simulink model "VCU_CS75_12_27_test_log"  (R2014a)
settings: Solver=FixedStepDiscrete  StartTime=0.0  StopTime=25  FixedStep=0.0005  RelTol=1e-3
undefined symbols (not defined in the file or in its folder): ecucoder_acal, ErrorSumMax1, ErrorSumMax2, ErrorSumMax3, I1, I2, I3, I_SW01_L, LaterlAngleCommand, LDW, Log_ErrorSumMax1, Log_ErrorSumMax2, Log_I1, Log_I2, Log_P1, Log_P2, Log_Takeover, P1, P2, P3, RemoteAcc, RemoteAcclPosition
libraries: simulink x927, ec5744lib x40
(part 21 of 31)

== system VCU_CS75_12_27_test_log/长安CS75底盘程序，20ms一次/Output/Subsystem/TransmitMessages11/GW_LCDAL_2EA/LCDAL_SEAStatus ==
  LCDAL_SEAStatus : Inport
  Constant{1..2,4..8} (7 alike) : Constant  Value=0  OutDataTypeStr=uint8
  LCDAL_SEAStatusRon : Rounding  Operator=round
  LCDAL_SEAStatus_1sat : Saturate  UpperLimit=192  LowerLimit=0
  LCDAL_SEAStatus_Convert : DataTypeConversion  OutDataTypeStr=uint8
  LCDAL_SEAStatus_Convert1 : DataTypeConversion  OutDataTypeStr=uint32
  LCDAL_SEAStatus_D : Product  Inputs=*/
  LCDAL_SEAStatus_F : Constant  OutDataTypeStr=single
  LCDAL_SEAStatus_L : simulink/Logic and Bit Operations/Bitwise Operator  logicop=AND  UseBitMask=on  BitMask=192  BitMaskRealWorld=Stored Integer
  LCDAL_SEAStatus_O : Constant  Value=0  OutDataTypeStr=single
  LCDAL_SEAStatus_S : ArithShift  BitShiftNumber=-6
  LCDAL_SEAStatus_sat : Saturate  UpperLimit=3  LowerLimit=0
  LCDAL_SEAStatus_st : Sum  Inputs=+-
  output1 : Outport
  output2 : Outport  Port=2
  output3 : Outport  Port=3
  output4 : Outport  Port=4
  output5 : Outport  Port=5
  output6 : Outport  Port=6
  output7 : Outport  Port=7
  output8 : Outport  Port=8
  wires:
  Constant8/1 -> output8/1
  Constant7/1 -> output7/1
  Constant6/1 -> output6/1
  Constant5/1 -> output5/1
  Constant4/1 -> output4/1
  Constant2/1 -> output2/1
  Constant1/1 -> output1/1
  LCDAL_SEAStatus_Convert/1 -> output3/1
  LCDAL_SEAStatus_L/1 -> LCDAL_SEAStatus_Convert/1
  LCDAL_SEAStatus_Convert1/1 -> LCDAL_SEAStatus_L/1
  LCDAL_SEAStatus_1sat/1 -> LCDAL_SEAStatus_Convert1/1
  LCDAL_SEAStatus_S/1 -> LCDAL_SEAStatus_1sat/1
  LCDAL_SEAStatusRon/1 -> LCDAL_SEAStatus_S/1
  LCDAL_SEAStatus_D/1 -> LCDAL_SEAStatusRon/1
  LCDAL_SEAStatus_F/1 -> LCDAL_SEAStatus_D/2
  LCDAL_SEAStatus_st/1 -> LCDAL_SEAStatus_D/1
  LCDAL_SEAStatus_O/1 -> LCDAL_SEAStatus_st/2
  LCDAL_SEAStatus_sat/1 -> LCDAL_SEAStatus_st/1
  LCDAL_SEAStatus/1 -> LCDAL_SEAStatus_sat/1

== system VCU_CS75_12_27_test_log/长安CS75底盘程序，20ms一次/Output/Subsystem/TransmitMessages11/GW_LCDAL_2EA/LCDAL_SystemStatus ==
  LCDAL_SystemStatus : Inport
  Constant{1,3..8} (7 alike) : Constant  Value=0  OutDataTypeStr=uint8
  LCDAL_SystemStatusRon : Rounding  Operator=round
  LCDAL_SystemStatus_1sat : Saturate  UpperLimit=224  LowerLimit=0
  LCDAL_SystemStatus_Convert : DataTypeConversion  OutDataTypeStr=uint8
  LCDAL_SystemStatus_Convert1 : DataTypeConversion  OutDataTypeStr=uint32
  LCDAL_SystemStatus_D : Product  Inputs=*/
  LCDAL_SystemStatus_F : Constant  OutDataTypeStr=single
  LCDAL_SystemStatus_L : simulink/Logic and Bit Operations/Bitwise Operator  logicop=AND  UseBitMask=on  BitMask=224  BitMaskRealWorld=Stored Integer
  LCDAL_SystemStatus_O : Constant  Value=0  OutDataTypeStr=single
  LCDAL_SystemStatus_S : ArithShift  BitShiftNumber=-5
  LCDAL_SystemStatus_sat : Saturate  UpperLimit=7  LowerLimit=0
  LCDAL_SystemStatus_st : Sum  Inputs=+-
  output1 : Outport
  output2 : Outport  Port=2
  output3 : Outport  Port=3
  output4 : Outport  Port=4
  output5 : Outport  Port=5
  output6 : Outport  Port=6
  output7 : Outport  Port=7
  output8 : Outport  Port=8
  wires:
  Constant8/1 -> output8/1
  Constant7/1 -> output7/1
  Constant6/1 -> output6/1
  Constant5/1 -> output5/1
  Constant4/1 -> output4/1
  Constant3/1 -> output3/1
  Constant1/1 -> output1/1
  LCDAL_SystemStatus_Convert/1 -> output2/1
  LCDAL_SystemStatus_L/1 -> LCDAL_SystemStatus_Convert/1
  LCDAL_SystemStatus_Convert1/1 -> LCDAL_SystemStatus_L/1
  LCDAL_SystemStatus_1sat/1 -> LCDAL_SystemStatus_Convert1/1
  LCDAL_SystemStatus_S/1 -> LCDAL_SystemStatus_1sat/1
  LCDAL_SystemStatusRon/1 -> LCDAL_SystemStatus_S/1
  LCDAL_SystemStatus_D/1 -> LCDAL_SystemStatusRon/1
  LCDAL_SystemStatus_F/1 -> LCDAL_SystemStatus_D/2
  LCDAL_SystemStatus_st/1 -> LCDAL_SystemStatus_D/1
  LCDAL_SystemStatus_O/1 -> LCDAL_SystemStatus_st/2
  LCDAL_SystemStatus_sat/1 -> LCDAL_SystemStatus_st/1
  LCDAL_SystemStatus/1 -> LCDAL_SystemStatus_sat/1

== system VCU_CS75_12_27_test_log/长安CS75底盘程序，20ms一次/Output/Subsystem/TransmitMessages13/GW_LCDAR_2FA/LCDAR_BSDLCAAlert ==
  LCDAR_BSDLCAAlert : Inport
  Constant{2..8} (7 alike) : Constant  Value=0  OutDataTypeStr=uint8
  LCDAR_BSDLCAAlertRon : Rounding  Operator=round
  LCDAR_BSDLCAAlert_1sat : Saturate  UpperLimit=48  LowerLimit=0
  LCDAR_BSDLCAAlert_Convert : DataTypeConversion  OutDataTypeStr=uint8
  LCDAR_BSDLCAAlert_Convert1 : DataTypeConversion  OutDataTypeStr=uint32
  LCDAR_BSDLCAAlert_D : Product  Inputs=*/
  LCDAR_BSDLCAAlert_F : Constant  OutDataTypeStr=single
  LCDAR_BSDLCAAlert_L : simulink/Logic and Bit Operations/Bitwise Operator  logicop=AND  UseBitMask=on  BitMask=48  BitMaskRealWorld=Stored Integer
  LCDAR_BSDLCAAlert_O : Constant  Value=0  OutDataTypeStr=single
  LCDAR_BSDLCAAlert_S : ArithShift  BitShiftNumber=-4
  LCDAR_BSDLCAAlert_sat : Saturate  UpperLimit=3  LowerLimit=0
  LCDAR_BSDLCAAlert_st : Sum  Inputs=+-
  output1 : Outport
  output2 : Outport  Port=2
  output3 : Outport  Port=3
  output4 : Outport  Port=4
  output5 : Outport  Port=5
  output6 : Outport  Port=6
  output7 : Outport  Port=7
  output8 : Outport  Port=8
  wires:
  LCDAR_BSDLCAAlert/1 -> LCDAR_BSDLCAAlert_sat/1
  LCDAR_BSDLCAAlert_sat/1 -> LCDAR_BSDLCAAlert_st/1
  LCDAR_BSDLCAAlert_O/1 -> LCDAR_BSDLCAAlert_st/2
  LCDAR_BSDLCAAlert_st/1 -> LCDAR_BSDLCAAlert_D/1
  LCDAR_BSDLCAAlert_F/1 -> LCDAR_BSDLCAAlert_D/2
  LCDAR_BSDLCAAlert_D/1 -> LCDAR_BSDLCAAlertRon/1
  LCDAR_BSDLCAAlertRon/1 -> LCDAR_BSDLCAAlert_S/1
  LCDAR_BSDLCAAlert_S/1 -> LCDAR_BSDLCAAlert_1sat/1
  LCDAR_BSDLCAAlert_1sat/1 -> LCDAR_BSDLCAAlert_Convert1/1
  LCDAR_BSDLCAAlert_Convert1/1 -> LCDAR_BSDLCAAlert_L/1
  LCDAR_BSDLCAAlert_L/1 -> LCDAR_BSDLCAAlert_Convert/1
  LCDAR_BSDLCAAlert_Convert/1 -> output1/1
  Constant2/1 -> output2/1
  Constant3/1 -> output3/1
  Constant4/1 -> output4/1
  Constant5/1 -> output5/1
  Constant6/1 -> output6/1
  Constant7/1 -> output7/1
  Constant8/1 -> output8/1

== system VCU_CS75_12_27_test_log/长安CS75底盘程序，20ms一次/Output/Subsystem/TransmitMessages13/GW_LCDAR_2FA/LCDAR_BSDLCAStatus ==
  LCDAR_BSDLCAStatus : Inport
  Constant{1,3..8} (7 alike) : Constant  Value=0  OutDataTypeStr=uint8
  LCDAR_BSDLCAStatusRon : Rounding  Operator=round
  LCDAR_BSDLCAStatus_1sat : Saturate  UpperLimit=24  LowerLimit=0
  LCDAR_BSDLCAStatus_Convert : DataTypeConversion  OutDataTypeStr=uint8
  LCDAR_BSDLCAStatus_Convert1 : DataTypeConversion  OutDataTypeStr=uint32
  LCDAR_BSDLCAStatus_D : Product  Inputs=*/
  LCDAR_BSDLCAStatus_F : Constant  OutDataTypeStr=single
  LCDAR_BSDLCAStatus_L : simulink/Logic and Bit Operations/Bitwise Operator  logicop=AND  UseBitMask=on  BitMask=24  BitMaskRealWorld=Stored Integer
  LCDAR_BSDLCAStatus_O : Constant  Value=0  OutDataTypeStr=single
  LCDAR_BSDLCAStatus_S : ArithShift  BitShiftNumber=-3
  LCDAR_BSDLCAStatus_sat : Saturate  UpperLimit=3  LowerLimit=0
  LCDAR_BSDLCAStatus_st : Sum  Inputs=+-
  output1 : Outport
  output2 : Outport  Port=2
  output3 : Outport  Port=3
  output4 : Outport  Port=4
  output5 : Outport  Port=5
  output6 : Outport  Port=6
  output7 : Outport  Port=7
  output8 : Outport  Port=8
  wires:
  LCDAR_BSDLCAStatus/1 -> LCDAR_BSDLCAStatus_sat/1
  LCDAR_BSDLCAStatus_sat/1 -> LCDAR_BSDLCAStatus_st/1
  LCDAR_BSDLCAStatus_O/1 -> LCDAR_BSDLCAStatus_st/2
  LCDAR_BSDLCAStatus_st/1 -> LCDAR_BSDLCAStatus_D/1
  LCDAR_BSDLCAStatus_F/1 -> LCDAR_BSDLCAStatus_D/2
  LCDAR_BSDLCAStatus_D/1 -> LCDAR_BSDLCAStatusRon/1
  LCDAR_BSDLCAStatusRon/1 -> LCDAR_BSDLCAStatus_S/1
  LCDAR_BSDLCAStatus_S/1 -> LCDAR_BSDLCAStatus_1sat/1
  LCDAR_BSDLCAStatus_1sat/1 -> LCDAR_BSDLCAStatus_Convert1/1
  LCDAR_BSDLCAStatus_Convert1/1 -> LCDAR_BSDLCAStatus_L/1
  LCDAR_BSDLCAStatus_L/1 -> LCDAR_BSDLCAStatus_Convert/1
  LCDAR_BSDLCAStatus_Convert/1 -> output2/1
  Constant1/1 -> output1/1
  Constant3/1 -> output3/1
  Constant4/1 -> output4/1
  Constant5/1 -> output5/1
  Constant6/1 -> output6/1
  Constant7/1 -> output7/1
  Constant8/1 -> output8/1

== system VCU_CS75_12_27_test_log/长安CS75底盘程序，20ms一次/Output/Subsystem/TransmitMessages13/GW_LCDAR_2FA/LCDAR_CTAAlert ==
  LCDAR_CTAAlert : Inport
  Constant{2..8} (7 alike) : Constant  Value=0  OutDataTypeStr=uint8
  LCDAR_CTAAlertABS : Abs
  LCDAR_CTAAlertCS : ArithShift  BitShiftNumber=-2
  LCDAR_CTAAlertConS : Constant  OutDataTypeStr=single
  LCDAR_CTAAlertCosR : Constant  Value=0  OutDataTypeStr=uint8
  LCDAR_CTAAlertROP : RelationalOperator  Operator=<  OutDataTypeStr=boolean
  LCDAR_CTAAlertRon : Rounding  Operator=round
  LCDAR_CTAAlertSW : Switch  Criteria=u2 ~= 0
  LCDAR_CTAAlert_1sat : Saturate  UpperLimit=3  LowerLimit=0
  LCDAR_CTAAlert_Convert : DataTypeConversion  OutDataTypeStr=uint8
  LCDAR_CTAAlert_Convert1 : DataTypeConversion  OutDataTypeStr=uint32
  LCDAR_CTAAlert_D : Product  Inputs=*/
  LCDAR_CTAAlert_F : Constant  OutDataTypeStr=single
  LCDAR_CTAAlert_L : simulink/Logic and Bit Operations/Bitwise Operator  logicop=AND  UseBitMask=on  BitMask=3  BitMaskRealWorld=Stored Integer
  LCDAR_CTAAlert_O : Constant  Value=0  OutDataTypeStr=single
  LCDAR_CTAAlert_S : ArithShift
  LCDAR_CTAAlert_sat : Saturate  UpperLimit=3  LowerLimit=0
  LCDAR_CTAAlert_st : Sum  Inputs=+-
  LCDAR_CTAAlertsubcon : Sum  Inputs=+-
  output1 : Outport
  output2 : Outport  Port=2
  output3 : Outport  Port=3
  output4 : Outport  Port=4
  output5 : Outport  Port=5
  output6 : Outport  Port=6
  output7 : Outport  Port=7
  output8 : Outport  Port=8
  wires:
  LCDAR_CTAAlert/1 -> LCDAR_CTAAlert_sat/1
  LCDAR_CTAAlert_sat/1 -> LCDAR_CTAAlert_st/1
  LCDAR_CTAAlert_O/1 -> LCDAR_CTAAlert_st/2
  LCDAR_CTAAlert_st/1 -> LCDAR_CTAAlert_D/1
  LCDAR_CTAAlert_F/1 -> LCDAR_CTAAlert_D/2
  LCDAR_CTAAlert_D/1 -> LCDAR_CTAAlertRon/1
  LCDAR_CTAAlertRon/1 -> LCDAR_CTAAlertROP/1, LCDAR_CTAAlertABS/1, LCDAR_CTAAlertSW/3
  LCDAR_CTAAlertCosR/1 -> LCDAR_CTAAlertROP/2
  LCDAR_CTAAlertConS/1 -> LCDAR_CTAAlertCS/1
  LCDAR_CTAAlertCS/1 -> LCDAR_CTAAlertsubcon/1
  LCDAR_CTAAlertABS/1 -> LCDAR_CTAAlertsubcon/2
  LCDAR_CTAAlertsubcon/1 -> LCDAR_CTAAlertSW/1
  LCDAR_CTAAlertROP/1 -> LCDAR_CTAAlertSW/2
  LCDAR_CTAAlertSW/1 -> LCDAR_CTAAlert_S/1
  LCDAR_CTAAlert_S/1 -> LCDAR_CTAAlert_1sat/1
  LCDAR_CTAAlert_1sat/1 -> LCDAR_CTAAlert_Convert1/1
  LCDAR_CTAAlert_Convert1/1 -> LCDAR_CTAAlert_L/1
  LCDAR_CTAAlert_L/1 -> LCDAR_CTAAlert_Convert/1
  LCDAR_CTAAlert_Convert/1 -> output1/1
  Constant2/1 -> output2/1
  Constant3/1 -> output3/1
  Constant4/1 -> output4/1
  Constant5/1 -> output5/1
  Constant6/1 -> output6/1
  Constant7/1 -> output7/1
  Constant8/1 -> output8/1

== system VCU_CS75_12_27_test_log/长安CS75底盘程序，20ms一次/Output/Subsystem/TransmitMessages13/GW_LCDAR_2FA/LCDAR_CTAStatus ==
  LCDAR_CTAStatus : Inport
  Constant{1,3..8} (7 alike) : Constant  Value=0  OutDataTypeStr=uint8
  LCDAR_CTAStatusRon : Rounding  Operator=round
  LCDAR_CTAStatus_1sat : Saturate  UpperLimit=6  LowerLimit=0
  LCDAR_CTAStatus_Convert : DataTypeConversion  OutDataTypeStr=uint8
  LCDAR_CTAStatus_Convert1 : DataTypeConversion  OutDataTypeStr=uint32
  LCDAR_CTAStatus_D : Product  Inputs=*/
  LCDAR_CTAStatus_F : Constant  OutDataTypeStr=single
  LCDAR_CTAStatus_L : simulink/Logic and Bit Operations/Bitwise Operator  logicop=AND  UseBitMask=on  BitMask=6  BitMaskRealWorld=Stored Integer
  LCDAR_CTAStatus_O : Constant  Value=0  OutDataTypeStr=single
  LCDAR_CTAStatus_S : ArithShift  BitShiftNumber=-1
  LCDAR_CTAStatus_sat : Saturate  UpperLimit=3  LowerLimit=0
  LCDAR_CTAStatus_st : Sum  Inputs=+-
  output1 : Outport
  output2 : Outport  Port=2
  output3 : Outport  Port=3
  output4 : Outport  Port=4
  output5 : Outport  Port=5
  output6 : Outport  Port=6
  output7 : Outport  Port=7
  output8 : Outport  Port=8
  wires:
  LCDAR_CTAStatus/1 -> LCDAR_CTAStatus_sat/1
  LCDAR_CTAStatus_sat/1 -> LCDAR_CTAStatus_st/1
  LCDAR_CTAStatus_O/1 -> LCDAR_CTAStatus_st/2
  LCDAR_CTAStatus_st/1 -> LCDAR_CTAStatus_D/1
  LCDAR_CTAStatus_F/1 -> LCDAR_CTAStatus_D/2
  LCDAR_CTAStatus_D/1 -> LCDAR_CTAStatusRon/1
  LCDAR_CTAStatusRon/1 -> LCDAR_CTAStatus_S/1
  LCDAR_CTAStatus_S/1 -> LCDAR_CTAStatus_1sat/1
  LCDAR_CTAStatus_1sat/1 -> LCDAR_CTAStatus_Convert1/1
  LCDAR_CTAStatus_Convert1/1 -> LCDAR_CTAStatus_L/1
  LCDAR_CTAStatus_L/1 -> LCDAR_CTAStatus_Convert/1
  LCDAR_CTAStatus_Convert/1 -> output2/1
  Constant1/1 -> output1/1
  Constant3/1 -> output3/1
  Constant4/1 -> output4/1
  Constant5/1 -> output5/1
  Constant6/1 -> output6/1
  Constant7/1 -> output7/1
  Constant8/1 -> output8/1

== system VCU_CS75_12_27_test_log/长安CS75底盘程序，20ms一次/Output/Subsystem/TransmitMessages13/GW_LCDAR_2FA/LCDAR_RCWAlert ==
  LCDAR_RCWAlert : Inport
  Constant{1..2,4..8} (7 alike) : Constant  Value=0  OutDataTypeStr=uint8
  LCDAR_RCWAlertRon : Rounding  Operator=round
  LCDAR_RCWAlert_1sat : Saturate  UpperLimit=3  LowerLimit=0
  LCDAR_RCWAlert_Convert : DataTypeConversion  OutDataTypeStr=uint8
  LCDAR_RCWAlert_Convert1 : DataTypeConversion  OutDataTypeStr=uint32
  LCDAR_RCWAlert_D : Product  Inputs=*/
  LCDAR_RCWAlert_F : Constant  OutDataTypeStr=single
  LCDAR_RCWAlert_L : simulink/Logic and Bit Operations/Bitwise Operator  logicop=AND  UseBitMask=on  BitMask=3  BitMaskRealWorld=Stored Integer
  LCDAR_RCWAlert_O : Constant  Value=0  OutDataTypeStr=single
  LCDAR_RCWAlert_S : ArithShift
  LCDAR_RCWAlert_sat : Saturate  UpperLimit=3  LowerLimit=0
  LCDAR_RCWAlert_st : Sum  Inputs=+-
  output1 : Outport
  output2 : Outport  Port=2
  output3 : Outport  Port=3
  output4 : Outport  Port=4
  output5 : Outport  Port=5
  output6 : Outport  Port=6
  output7 : Outport  Port=7
  output8 : Outport  Port=8
  wires:
  LCDAR_RCWAlert/1 -> LCDAR_RCWAlert_sat/1
  LCDAR_RCWAlert_sat/1 -> LCDAR_RCWAlert_st/1
  LCDAR_RCWAlert_O/1 -> LCDAR_RCWAlert_st/2
  LCDAR_RCWAlert_st/1 -> LCDAR_RCWAlert_D/1
  LCDAR_RCWAlert_F/1 -> LCDAR_RCWAlert_D/2
  LCDAR_RCWAlert_D/1 -> LCDAR_RCWAlertRon/1
  LCDAR_RCWAlertRon/1 -> LCDAR_RCWAlert_S/1
  LCDAR_RCWAlert_S/1 -> LCDAR_RCWAlert_1sat/1
  LCDAR_RCWAlert_1sat/1 -> LCDAR_RCWAlert_Convert1/1
  LCDAR_RCWAlert_Convert1/1 -> LCDAR_RCWAlert_L/1
  LCDAR_RCWAlert_L/1 -> LCDAR_RCWAlert_Convert/1
  LCDAR_RCWAlert_Convert/1 -> output3/1
  Constant1/1 -> output1/1
  Constant2/1 -> output2/1
  Constant4/1 -> output4/1
  Constant5/1 -> output5/1
  Constant6/1 -> output6/1
  Constant7/1 -> output7/1
  Constant8/1 -> output8/1

== system VCU_CS75_12_27_test_log/长安CS75底盘程序，20ms一次/Output/Subsystem/TransmitMessages13/GW_LCDAR_2FA/LCDAR_RCWStatus ==
  LCDAR_RCWStatus : Inport
  Constant{1..3,5..8} (7 alike) : Constant  Value=0  OutDataTypeStr=uint8
  LCDAR_RCWStatusRon : Rounding  Operator=round
  LCDAR_RCWStatus_1sat : Saturate  UpperLimit=48  LowerLimit=0
  LCDAR_RCWStatus_Convert : DataTypeConversion  OutDataTypeStr=uint8
  LCDAR_RCWStatus_Convert1 : DataTypeConversion  OutDataTypeStr=uint32
  LCDAR_RCWStatus_D : Product  Inputs=*/
  LCDAR_RCWStatus_F : Constant  OutDataTypeStr=single
  LCDAR_RCWStatus_L : simulink/Logic and Bit Operations/Bitwise Operator  logicop=AND  UseBitMask=on  BitMask=48  BitMaskRealWorld=Stored Integer
  LCDAR_RCWStatus_O : Constant  Value=0  OutDataTypeStr=single
  LCDAR_RCWStatus_S : ArithShift  BitShiftNumber=-4
  LCDAR_RCWStatus_sat : Saturate  UpperLimit=3  LowerLimit=0
  LCDAR_RCWStatus_st : Sum  Inputs=+-
  output1 : Outport
  output2 : Outport  Port=2
  output3 : Outport  Port=3
  output4 : Outport  Port=4
  output5 : Outport  Port=5
  output6 : Outport  Port=6
  output7 : Outport  Port=7
  output8 : Outport  Port=8
  wires:
  LCDAR_RCWStatus/1 -> LCDAR_RCWStatus_sat/1
  LCDAR_RCWStatus_sat/1 -> LCDAR_RCWStatus_st/1
  LCDAR_RCWStatus_O/1 -> LCDAR_RCWStatus_st/2
  LCDAR_RCWStatus_st/1 -> LCDAR_RCWStatus_D/1
  LCDAR_RCWStatus_F/1 -> LCDAR_RCWStatus_D/2
  LCDAR_RCWStatus_D/1 -> LCDAR_RCWStatusRon/1
  LCDAR_RCWStatusRon/1 -> LCDAR_RCWStatus_S/1
  LCDAR_RCWStatus_S/1 -> LCDAR_RCWStatus_1sat/1
  LCDAR_RCWStatus_1sat/1 -> LCDAR_RCWStatus_Convert1/1
  LCDAR_RCWStatus_Convert1/1 -> LCDAR_RCWStatus_L/1
  LCDAR_RCWStatus_L/1 -> LCDAR_RCWStatus_Convert/1
  LCDAR_RCWStatus_Convert/1 -> output4/1
  Constant1/1 -> output1/1
  Constant2/1 -> output2/1
  Constant3/1 -> output3/1
  Constant5/1 -> output5/1
  Constant6/1 -> output6/1
  Constant7/1 -> output7/1
  Constant8/1 -> output8/1

== system VCU_CS75_12_27_test_log/长安CS75底盘程序，20ms一次/Output/Subsystem/TransmitMessages13/GW_LCDAR_2FA/LCDAR_SEAAlert ==
  LCDAR_SEAAlert : Inport
  Constant{2..8} (7 alike) : Constant  Value=0  OutDataTypeStr=uint8
  LCDAR_SEAAlertRon : Rounding  Operator=round
  LCDAR_SEAAlert_1sat : Saturate  UpperLimit=12  LowerLimit=0
  LCDAR_SEAAlert_Convert : DataTypeConversion  OutDataTypeStr=uint8
  LCDAR_SEAAlert_Convert1 : DataTypeConversion  OutDataTypeStr=uint32
  LCDAR_SEAAlert_D : Product  Inputs=*/
  LCDAR_SEAAlert_F : Constant  OutDataTypeStr=single
  LCDAR_SEAAlert_L : simulink/Logic and Bit Operations/Bitwise Operator  logicop=AND  UseBitMask=on  BitMask=12  BitMaskRealWorld=Stored Integer
  LCDAR_SEAAlert_O : Constant  Value=0  OutDataTypeStr=single
  LCDAR_SEAAlert_S : ArithShift  BitShiftNumber=-2
  LCDAR_SEAAlert_sat : Saturate  UpperLimit=3  LowerLimit=0
  LCDAR_SEAAlert_st : Sum  Inputs=+-
  output1 : Outport
  output2 : Outport  Port=2
  output3 : Outport  Port=3
  output4 : Outport  Port=4
  output5 : Outport  Port=5
  output6 : Outport  Port=6
  output7 : Outport  Port=7
  output8 : Outport  Port=8
  wires:
  LCDAR_SEAAlert/1 -> LCDAR_SEAAlert_sat/1
  LCDAR_SEAAlert_sat/1 -> LCDAR_SEAAlert_st/1
  LCDAR_SEAAlert_O/1 -> LCDAR_SEAAlert_st/2
  LCDAR_SEAAlert_st/1 -> LCDAR_SEAAlert_D/1
  LCDAR_SEAAlert_F/1 -> LCDAR_SEAAlert_D/2
  LCDAR_SEAAlert_D/1 -> LCDAR_SEAAlertRon/1
  LCDAR_SEAAlertRon/1 -> LCDAR_SEAAlert_S/1
  LCDAR_SEAAlert_S/1 -> LCDAR_SEAAlert_1sat/1
  LCDAR_SEAAlert_1sat/1 -> LCDAR_SEAAlert_Convert1/1
  LCDAR_SEAAlert_Convert1/1 -> LCDAR_SEAAlert_L/1
  LCDAR_SEAAlert_L/1 -> LCDAR_SEAAlert_Convert/1
  LCDAR_SEAAlert_Convert/1 -> output1/1
  Constant2/1 -> output2/1
  Constant3/1 -> output3/1
  Constant4/1 -> output4/1
  Constant5/1 -> output5/1
  Constant6/1 -> output6/1
  Constant7/1 -> output7/1
  Constant8/1 -> output8/1

== system VCU_CS75_12_27_test_log/长安CS75底盘程序，20ms一次/Output/Subsystem/TransmitMessages13/GW_LCDAR_2FA/LCDAR_SEAStatus ==
  LCDAR_SEAStatus : Inport
  Constant{1..2,4..8} (7 alike) : Constant  Value=0  OutDataTypeStr=uint8
  LCDAR_SEAStatusRon : Rounding  Operator=round
  LCDAR_SEAStatus_1sat : Saturate  UpperLimit=48  LowerLimit=0
  LCDAR_SEAStatus_Convert : DataTypeConversion  OutDataTypeStr=uint8
  LCDAR_SEAStatus_Convert1 : DataTypeConversion  OutDataTypeStr=uint32
  LCDAR_SEAStatus_D : Product  Inputs=*/
  LCDAR_SEAStatus_F : Constant  OutDataTypeStr=single
  LCDAR_SEAStatus_L : simulink/Logic and Bit Operations/Bitwise Operator  logicop=AND  UseBitMask=on  BitMask=48  BitMaskRealWorld=Stored Integer
  LCDAR_SEAStatus_O : Constant  Value=0  OutDataTypeStr=single
  LCDAR_SEAStatus_S : ArithShift  BitShiftNumber=-4
  LCDAR_SEAStatus_sat : Saturate  UpperLimit=3  LowerLimit=0
  LCDAR_SEAStatus_st : Sum  Inputs=+-
  output1 : Outport
  output2 : Outport  Port=2
  output3 : Outport  Port=3
  output4 : Outport  Port=4
  output5 : Outport  Port=5
  output6 : Outport  Port=6
  output7 : Outport  Port=7
  output8 : Outport  Port=8
  wires:
  LCDAR_SEAStatus/1 -> LCDAR_SEAStatus_sat/1
  LCDAR_SEAStatus_sat/1 -> LCDAR_SEAStatus_st/1
  LCDAR_SEAStatus_O/1 -> LCDAR_SEAStatus_st/2
  LCDAR_SEAStatus_st/1 -> LCDAR_SEAStatus_D/1
  LCDAR_SEAStatus_F/1 -> LCDAR_SEAStatus_D/2
  LCDAR_SEAStatus_D/1 -> LCDAR_SEAStatusRon/1
  LCDAR_SEAStatusRon/1 -> LCDAR_SEAStatus_S/1
  LCDAR_SEAStatus_S/1 -> LCDAR_SEAStatus_1sat/1
  LCDAR_SEAStatus_1sat/1 -> LCDAR_SEAStatus_Convert1/1
  LCDAR_SEAStatus_Convert1/1 -> LCDAR_SEAStatus_L/1
  LCDAR_SEAStatus_L/1 -> LCDAR_SEAStatus_Convert/1
  LCDAR_SEAStatus_Convert/1 -> output3/1
  Constant1/1 -> output1/1
  Constant2/1 -> output2/1
  Constant4/1 -> output4/1
  Constant5/1 -> output5/1
  Constant6/1 -> output6/1
  Constant7/1 -> output7/1
  Constant8/1 -> output8/1

== system VCU_CS75_12_27_test_log/长安CS75底盘程序，20ms一次/Output/Subsystem/TransmitMessages13/GW_LCDAR_2FA/LCDAR_SystemStatus ==
  LCDAR_SystemStatus : Inport
  Constant{1,3..8} (7 alike) : Constant  Value=0  OutDataTypeStr=uint8
  LCDAR_SystemStatusRon : Rounding  Operator=round
  LCDAR_SystemStatus_1sat : Saturate  UpperLimit=224  LowerLimit=0
  LCDAR_SystemStatus_Convert : DataTypeConversion  OutDataTypeStr=uint8
  LCDAR_SystemStatus_Convert1 : DataTypeConversion  OutDataTypeStr=uint32
  LCDAR_SystemStatus_D : Product  Inputs=*/
  LCDAR_SystemStatus_F : Constant  OutDataTypeStr=single
  LCDAR_SystemStatus_L : simulink/Logic and Bit Operations/Bitwise Operator  logicop=AND  UseBitMask=on  BitMask=224  BitMaskRealWorld=Stored Integer
  LCDAR_SystemStatus_O : Constant  Value=0  OutDataTypeStr=single
  LCDAR_SystemStatus_S : ArithShift  BitShiftNumber=-5
  LCDAR_SystemStatus_sat : Saturate  UpperLimit=7  LowerLimit=0
  LCDAR_SystemStatus_st : Sum  Inputs=+-
  output1 : Outport
  output2 : Outport  Port=2
  output3 : Outport  Port=3
  output4 : Outport  Port=4
  output5 : Outport  Port=5
  output6 : Outport  Port=6
  output7 : Outport  Port=7
  output8 : Outport  Port=8
  wires:
  LCDAR_SystemStatus/1 -> LCDAR_SystemStatus_sat/1
  LCDAR_SystemStatus_sat/1 -> LCDAR_SystemStatus_st/1
  LCDAR_SystemStatus_O/1 -> LCDAR_SystemStatus_st/2
  LCDAR_SystemStatus_st/1 -> LCDAR_SystemStatus_D/1
  LCDAR_SystemStatus_F/1 -> LCDAR_SystemStatus_D/2
  LCDAR_SystemStatus_D/1 -> LCDAR_SystemStatusRon/1
  LCDAR_SystemStatusRon/1 -> LCDAR_SystemStatus_S/1
  LCDAR_SystemStatus_S/1 -> LCDAR_SystemStatus_1sat/1
  LCDAR_SystemStatus_1sat/1 -> LCDAR_SystemStatus_Convert1/1
  LCDAR_SystemStatus_Convert1/1 -> LCDAR_SystemStatus_L/1
  LCDAR_SystemStatus_L/1 -> LCDAR_SystemStatus_Convert/1
  LCDAR_SystemStatus_Convert/1 -> output2/1
  Constant1/1 -> output1/1
  Constant3/1 -> output3/1
  Constant4/1 -> output4/1
  Constant5/1 -> output5/1
  Constant6/1 -> output6/1
  Constant7/1 -> output7/1
  Constant8/1 -> output8/1

== system VCU_CS75_12_27_test_log/长安CS75底盘程序，20ms一次/Output/Subsystem/TransmitMessages14/LAS_2AD/CRC ==
  CRC : Inport
  CRCRon : Rounding  Operator=round
  CRC_1sat : Saturate  UpperLimit=255  LowerLimit=0
  CRC_Convert : DataTypeConversion  OutDataTypeStr=uint8
  CRC_Convert1 : DataTypeConversion  OutDataTypeStr=uint32
  CRC_D : Product  Inputs=*/
  CRC_F : Constant  OutDataTypeStr=single
  CRC_L : simulink/Logic and Bit Operations/Bitwise Operator  logicop=AND  UseBitMask=on  BitMask=255  BitMaskRealWorld=Stored Integer
  CRC_O : Constant  Value=0  OutDataTypeStr=single
  CRC_S : ArithShift
  CRC_sat : Saturate  UpperLimit=0  LowerLimit=0
  CRC_st : Sum  Inputs=+-
  Constant{1..7} (7 alike) : Constant  Value=0  OutDataTypeStr=uint8
  output1 : Outport
  output2 : Outport  Port=2
  output3 : Outport  Port=3
  output4 : Outport  Port=4
  output5 : Outport  Port=5
  output6 : Outport  Port=6
  output7 : Outport  Port=7
  output8 : Outport  Port=8
  wires:
  Constant7/1 -> output7/1
  Constant6/1 -> output6/1
  Constant5/1 -> output5/1
  Constant4/1 -> output4/1
  Constant3/1 -> output3/1
  Constant2/1 -> output2/1
  Constant1/1 -> output1/1
  CRC_Convert/1 -> output8/1
  CRC_L/1 -> CRC_Convert/1
  CRC_Convert1/1 -> CRC_L/1
  CRC_1sat/1 -> CRC_Convert1/1
  CRC_S/1 -> CRC_1sat/1
  CRCRon/1 -> CRC_S/1
  CRC_D/1 -> CRCRon/1
  CRC_F/1 -> CRC_D/2
  CRC_st/1 -> CRC_D/1
  CRC_O/1 -> CRC_st/2
  CRC_sat/1 -> CRC_st/1
  CRC/1 -> CRC_sat/1

== system VCU_CS75_12_27_test_log/长安CS75底盘程序，20ms一次/Output/Subsystem/TransmitMessages14/LAS_2AD/LAS_DriverHandsOff ==
  LAS_DriverHandsOff : Inport
  Constant{1,3..8} (7 alike) : Constant  Value=0  OutDataTypeStr=uint8
  LAS_DriverHandsOffRon : Rounding  Operator=round
  LAS_DriverHandsOff_1sat : Saturate  UpperLimit=3  LowerLimit=0
  LAS_DriverHandsOff_Convert : DataTypeConversion  OutDataTypeStr=uint8
  LAS_DriverHandsOff_Convert1 : DataTypeConversion  OutDataTypeStr=uint32
  LAS_DriverHandsOff_D : Product  Inputs=*/
  LAS_DriverHandsOff_F : Constant  OutDataTypeStr=single
  LAS_DriverHandsOff_L : simulink/Logic and Bit Operations/Bitwise Operator  logicop=AND  UseBitMask=on  BitMask=3  BitMaskRealWorld=Stored Integer
  LAS_DriverHandsOff_O : Constant  Value=0  OutDataTypeStr=single
  LAS_DriverHandsOff_S : ArithShift
  LAS_DriverHandsOff_sat : Saturate  UpperLimit=3  LowerLimit=0
  LAS_DriverHandsOff_st : Sum  Inputs=+-
  output1 : Outport
  output2 : Outport  Port=2
  output3 : Outport  Port=3
  output4 : Outport  Port=4
  output5 : Outport  Port=5
  output6 : Outport  Port=6
  output7 : Outport  Port=7
  output8 : Outport  Port=8
  wires:
  Constant8/1 -> output8/1
  Constant7/1 -> output7/1
  Constant6/1 -> output6/1
  Constant5/1 -> output5/1
  Constant4/1 -> output4/1
  Constant3/1 -> output3/1
  Constant1/1 -> output1/1
  LAS_DriverHandsOff_Convert/1 -> output2/1
  LAS_DriverHandsOff_L/1 -> LAS_DriverHandsOff_Convert/1
  LAS_DriverHandsOff_Convert1/1 -> LAS_DriverHandsOff_L/1
  LAS_DriverHandsOff_1sat/1 -> LAS_DriverHandsOff_Convert1/1
  LAS_DriverHandsOff_S/1 -> LAS_DriverHandsOff_1sat/1
  LAS_DriverHandsOffRon/1 -> LAS_DriverHandsOff_S/1
  LAS_DriverHandsOff_D/1 -> LAS_DriverHandsOffRon/1
  LAS_DriverHandsOff_F/1 -> LAS_DriverHandsOff_D/2
  LAS_DriverHandsOff_st/1 -> LAS_DriverHandsOff_D/1
  LAS_DriverHandsOff_O/1 -> LAS_DriverHandsOff_st/2
  LAS_DriverHandsOff_sat/1 -> LAS_DriverHandsOff_st/1
  LAS_DriverHandsOff/1 -> LAS_DriverHandsOff_sat/1

== system VCU_CS75_12_27_test_log/长安CS75底盘程序，20ms一次/Output/Subsystem/TransmitMessages14/LAS_2AD/LAS_IACCMode ==
  LAS_IACCMode : Inport
  Constant{1..3,5..8} (7 alike) : Constant  Value=0  OutDataTypeStr=uint8
  LAS_IACCModeRon : Rounding  Operator=round
  LAS_IACCMode_1sat : Saturate  UpperLimit=7  LowerLimit=0
  LAS_IACCMode_Convert : DataTypeConversion  OutDataTypeStr=uint8
  LAS_IACCMode_Convert1 : DataTypeConversion  OutDataTypeStr=uint32
  LAS_IACCMode_D : Product  Inputs=*/
  LAS_IACCMode_F : Constant  OutDataTypeStr=single
  LAS_IACCMode_L : simulink/Logic and Bit Operations/Bitwise Operator  logicop=AND  UseBitMask=on  BitMask=7  BitMaskRealWorld=Stored Integer
  LAS_IACCMode_O : Constant  Value=0  OutDataTypeStr=single
  LAS_IACCMode_S : ArithShift
  LAS_IACCMode_sat : Saturate  UpperLimit=7  LowerLimit=0
  LAS_IACCMode_st : Sum  Inputs=+-
  output1 : Outport
  output2 : Outport  Port=2
  output3 : Outport  Port=3
  output4 : Outport  Port=4
  output5 : Outport  Port=5
  output6 : Outport  Port=6
  output7 : Outport  Port=7
  output8 : Outport  Port=8
  wires:
  Constant8/1 -> output8/1
  Constant7/1 -> output7/1
  Constant6/1 -> output6/1
  Constant5/1 -> output5/1
  Constant3/1 -> output3/1
  Constant2/1 -> output2/1
  Constant1/1 -> output1/1
  LAS_IACCMode_Convert/1 -> output4/1
  LAS_IACCMode_L/1 -> LAS_IACCMode_Convert/1
  LAS_IACCMode_Convert1/1 -> LAS_IACCMode_L/1
  LAS_IACCMode_1sat/1 -> LAS_IACCMode_Convert1/1
  LAS_IACCMode_S/1 -> LAS_IACCMode_1sat/1
  LAS_IACCModeRon/1 -> LAS_IACCMode_S/1
  LAS_IACCMode_D/1 -> LAS_IACCModeRon/1
  LAS_IACCMode_F/1 -> LAS_IACCMode_D/2
  LAS_IACCMode_st/1 -> LAS_IACCMode_D/1
  LAS_IACCMode_O/1 -> LAS_IACCMode_st/2
  LAS_IACCMode_sat/1 -> LAS_IACCMode_st/1
  LAS_IACCMode/1 -> LAS_IACCMode_sat/1

== system VCU_CS75_12_27_test_log/长安CS75底盘程序，20ms一次/Output/Subsystem/TransmitMessages14/LAS_2AD/LAS_IACCTextInfoForDriver ==
  LAS_IACCTextInfoForDriver : Inport
  Constant{1..3,5..8} (7 alike) : Constant  Value=0  OutDataTypeStr=uint8
  LAS_IACCTextInfoForDriverRon : Rounding  Operator=round
  LAS_IACCTextInfoForDriver_1sat : Saturate  UpperLimit=248  LowerLimit=0
  LAS_IACCTextInfoForDriver_Convert : DataTypeConversion  OutDataTypeStr=uint8
  LAS_IACCTextInfoForDriver_Convert1 : DataTypeConversion  OutDataTypeStr=uint32
  LAS_IACCTextInfoForDriver_D : Product  Inputs=*/
  LAS_IACCTextInfoForDriver_F : Constant  OutDataTypeStr=single
  LAS_IACCTextInfoForDriver_L : simulink/Logic and Bit Operations/Bitwise Operator  logicop=AND  UseBitMask=on  BitMask=248  BitMaskRealWorld=Stored Integer
  LAS_IACCTextInfoForDriver_O : Constant  Value=0  OutDataTypeStr=single
  LAS_IACCTextInfoForDriver_S : ArithShift  BitShiftNumber=-3
  LAS_IACCTextInfoForDriver_sat : Saturate  UpperLimit=0  LowerLimit=0
  LAS_IACCTextInfoForDriver_st : Sum  Inputs=+-
  output1 : Outport
  output2 : Outport  Port=2
  output3 : Outport  Port=3
  output4 : Outport  Port=4
  output5 : Outport  Port=5
  output6 : Outport  Port=6
  output7 : Outport  Port=7
  output8 : Outport  Port=8
  wires:
  Constant8/1 -> output8/1
  Constant7/1 -> output7/1
  Constant6/1 -> output6/1
  Constant5/1 -> output5/1
  Constant3/1 -> output3/1
  Constant2/1 -> output2/1
  Constant1/1 -> output1/1
  LAS_IACCTextInfoForDriver_Convert/1 -> output4/1
  LAS_IACCTextInfoForDriver_L/1 -> LAS_IACCTextInfoForDriver_Convert/1
  LAS_IACCTextInfoForDriver_Convert1/1 -> LAS_IACCTextInfoForDriver_L/1
  LAS_IACCTextInfoForDriver_1sat/1 -> LAS_IACCTextInfoForDriver_Convert1/1
  LAS_IACCTextInfoForDriver_S/1 -> LAS_IACCTextInfoForDriver_1sat/1
  LAS_IACCTextInfoForDriverRon/1 -> LAS_IACCTextInfoForDriver_S/1
  LAS_IACCTextInfoForDriver_D/1 -> LAS_IACCTextInfoForDriverRon/1
  LAS_IACCTextInfoForDriver_F/1 -> LAS_IACCTextInfoForDriver_D/2
  LAS_IACCTextInfoForDriver_st/1 -> LAS_IACCTextInfoForDriver_D/1
  LAS_IACCTextInfoForDriver_O/1 -> LAS_IACCTextInfoForDriver_st/2
  LAS_IACCTextInfoForDriver_sat/1 -> LAS_IACCTextInfoForDriver_st/1
  LAS_IACCTextInfoForDriver/1 -> LAS_IACCTextInfoForDriver_sat/1

== system VCU_CS75_12_27_test_log/长安CS75底盘程序，20ms一次/Output/Subsystem/TransmitMessages14/LAS_2AD/LAS_TargetBasedLateralCOntrol ==
  LAS_TargetBasedLateralCOntrol : Inport
  Constant{2..8} (7 alike) : Constant  Value=0  OutDataTypeStr=uint8
  LAS_TargetBasedLateralCOntrolRon : Rounding  Operator=round
  LAS_TargetBasedLateralCOntrol_1sat : Saturate  UpperLimit=3  LowerLimit=0
  LAS_TargetBasedLateralCOntrol_Convert : DataTypeConversion  OutDataTypeStr=uint8
  LAS_TargetBasedLateralCOntrol_Convert1 : DataTypeConversion  OutDataTypeStr=uint32
  LAS_TargetBasedLateralCOntrol_D : Product  Inputs=*/
  LAS_TargetBasedLateralCOntrol_F : Constant  OutDataTypeStr=single
  LAS_TargetBasedLateralCOntrol_L : simulink/Logic and Bit Operations/Bitwise Operator  logicop=AND  UseBitMask=on  BitMask=3  BitMaskRealWorld=Stored Integer
  LAS_TargetBasedLateralCOntrol_O : Constant  Value=0  OutDataTypeStr=single
  LAS_TargetBasedLateralCOntrol_S : ArithShift
  LAS_TargetBasedLateralCOntrol_sat : Saturate  UpperLimit=0  LowerLimit=0
  LAS_TargetBasedLateralCOntrol_st : Sum  Inputs=+-
  output1 : Outport
  output2 : Outport  Port=2
  output3 : Outport  Port=3
  output4 : Outport  Port=4
  output5 : Outport  Port=5
  output6 : Outport  Port=6
  output7 : Outport  Port=7
  output8 : Outport  Port=8
  wires:
  Constant8/1 -> output8/1
  Constant7/1 -> output7/1
  Constant6/1 -> output6/1
  Constant5/1 -> output5/1
  Constant4/1 -> output4/1
  Constant3/1 -> output3/1
  Constant2/1 -> output2/1
  LAS_TargetBasedLateralCOntrol_Convert/1 -> output1/1
  LAS_TargetBasedLateralCOntrol_L/1 -> LAS_TargetBasedLateralCOntrol_Convert/1
  LAS_TargetBasedLateralCOntrol_Convert1/1 -> LAS_TargetBasedLateralCOntrol_L/1
  LAS_TargetBasedLateralCOntrol_1sat/1 -> LAS_TargetBasedLateralCOntrol_Convert1/1
  LAS_TargetBasedLateralCOntrol_S/1 -> LAS_TargetBasedLateralCOntrol_1sat/1
  LAS_TargetBasedLateralCOntrolRon/1 -> LAS_TargetBasedLateralCOntrol_S/1
  LAS_TargetBasedLateralCOntrol_D/1 -> LAS_TargetBasedLateralCOntrolRon/1
  LAS_TargetBasedLateralCOntrol_F/1 -> LAS_TargetBasedLateralCOntrol_D/2
  LAS_TargetBasedLateralCOntrol_st/1 -> LAS_TargetBasedLateralCOntrol_D/1
  LAS_TargetBasedLateralCOntrol_O/1 -> LAS_TargetBasedLateralCOntrol_st/2
  LAS_TargetBasedLateralCOntrol_sat/1 -> LAS_TargetBasedLateralCOntrol_st/1
  LAS_TargetBasedLateralCOntrol/1 -> LAS_TargetBasedLateralCOntrol_sat/1

== system VCU_CS75_12_27_test_log/长安CS75底盘程序，20ms一次/Output/Subsystem/TransmitMessages14/LAS_2AD/RollingConter ==
  RollingConter : Inport
  Constant{1..6,8} (7 alike) : Constant  Value=0  OutDataTypeStr=uint8
  RollingConterRon : Rounding  Operator=round
  RollingConter_1sat : Saturate  UpperLimit=15  LowerLimit=0
  RollingConter_Convert : DataTypeConversion  OutDataTypeStr=uint8
  RollingConter_Convert1 : DataTypeConversion  OutDataTypeStr=uint32
  RollingConter_D : Product  Inputs=*/
  RollingConter_F : Constant  OutDataTypeStr=single
  RollingConter_L : simulink/Logic and Bit Operations/Bitwise Operator  logicop=AND  UseBitMask=on  BitMask=15  BitMaskRealWorld=Stored Integer
  RollingConter_O : Constant  Value=0  OutDataTypeStr=single
  RollingConter_S : ArithShift
  RollingConter_sat : Saturate  UpperLimit=0  LowerLimit=0
  RollingConter_st : Sum  Inputs=+-
  output1 : Outport
  output2 : Outport  Port=2
  output3 : Outport  Port=3
  output4 : Outport  Port=4
  output5 : Outport  Port=5
  output6 : Outport  Port=6
  output7 : Outport  Port=7
  output8 : Outport  Port=8
  wires:
  Constant8/1 -> output8/1
  Constant6/1 -> output6/1
  Constant5/1 -> output5/1
  Constant4/1 -> output4/1
  Constant3/1 -> output3/1
  Constant2/1 -> output2/1
  Constant1/1 -> output1/1
  RollingConter_Convert/1 -> output7/1
  RollingConter_L/1 -> RollingConter_Convert/1
  RollingConter_Convert1/1 -> RollingConter_L/1
  RollingConter_1sat/1 -> RollingConter_Convert1/1
  RollingConter_S/1 -> RollingConter_1sat/1
  RollingConterRon/1 -> RollingConter_S/1
  RollingConter_D/1 -> RollingConterRon/1
  RollingConter_F/1 -> RollingConter_D/2
  RollingConter_st/1 -> RollingConter_D/1
  RollingConter_O/1 -> RollingConter_st/2
  RollingConter_sat/1 -> RollingConter_st/1
  RollingConter/1 -> RollingConter_sat/1

== system VCU_CS75_12_27_test_log/长安CS75底盘程序，20ms一次/Output/Subsystem/TransmitMessages2/ACC_3C5/ACC_TargetRange ==
  ACC_TargetRange : Inport
  ACC_TargetRangeBitCov : DataTypeConversion  OutDataTypeStr=uint8
  ACC_TargetRangeCOV : DataTypeConversion  OutDataTypeStr=uint8
  ACC_TargetRangeRon : Rounding  Operator=round
  ACC_TargetRange_1sat : Saturate  UpperLimit=65408  LowerLimit=0
  ACC_TargetRange_And : simulink/Logic and Bit Operations/Bitwise Operator  logicop=AND  UseBitMask=off  NumInputPorts=2  BitMask=bin2dec('11011001')  BitMaskRealWorld=Stored Integer
  ACC_TargetRange_And_C : Constant  Value=255  OutDataTypeStr=uint32
  ACC_TargetRange_Convert : DataTypeConversion  OutDataTypeStr=uint32
  ACC_TargetRange_D : Product  Inputs=*/
  ACC_TargetRange_D1 : Product  Inputs=*/
  ACC_TargetRange_F : Constant  Value=0.5  OutDataTypeStr=single
  ACC_TargetRange_L : simulink/Logic and Bit Operations/Bitwise Operator  logicop=AND  UseBitMask=on  BitMask=65408  BitMaskRealWorld=Stored Integer
  ACC_TargetRange_O : Constant  Value=0  OutDataTypeStr=single
  ACC_TargetRange_S : ArithShift  BitShiftNumber=-7
  ACC_TargetRange_sat : Saturate  UpperLimit=250  LowerLimit=0
  ACC_TargetRange_st : Sum  Inputs=+-
  ACC_TargetRangeoutput2_C : Constant  Value=256
  Constant{1,4..8} (6 alike) : Constant  Value=0  OutDataTypeStr=uint8
  output1 : Outport
  output2 : Outport  Port=2
  output3 : Outport  Port=3
  output4 : Outport  Port=4
  output5 : Outport  Port=5
  output6 : Outport  Port=6
  output7 : Outport  Port=7
  output8 : Outport  Port=8
  wires:
  ACC_TargetRange/1 -> ACC_TargetRange_sat/1
  ACC_TargetRange_sat/1 -> ACC_TargetRange_st/1
  ACC_TargetRange_O/1 -> ACC_TargetRange_st/2
  ACC_TargetRange_st/1 -> ACC_TargetRange_D/1
  ACC_TargetRange_F/1 -> ACC_TargetRange_D/2
  ACC_TargetRange_D/1 -> ACC_TargetRangeRon/1
  ACC_TargetRangeRon/1 -> ACC_TargetRange_S/1
  ACC_TargetRange_S/1 -> ACC_TargetRange_1sat/1
  ACC_TargetRange_1sat/1 -> ACC_TargetRange_Convert/1
  ACC_TargetRange_Convert/1 -> ACC_TargetRange_L/1
  ACC_TargetRange_L/1 -> ACC_TargetRange_D1/1, ACC_TargetRange_And/1
  ACC_TargetRangeoutput2_C/1 -> ACC_TargetRange_D1/2
  ACC_TargetRange_D1/1 -> ACC_TargetRangeCOV/1
  ACC_TargetRangeCOV/1 -> output2/1
  ACC_TargetRange_And_C/1 -> ACC_TargetRange_And/2
  ACC_TargetRange_And/1 -> ACC_TargetRangeBitCov/1
  ACC_TargetRangeBitCov/1 -> output3/1
  Constant1/1 -> output1/1
  Constant4/1 -> output4/1
  Constant5/1 -> output5/1
  Constant6/1 -> output6/1
  Constant7/1 -> output7/1
  Constant8/1 -> output8/1

== system VCU_CS75_12_27_test_log/长安CS75底盘程序，20ms一次/Output/Subsystem/TransmitMessages2/ACC_3C5/ACC_TargetType ==
  ACC_TargetType : Inport
  ACC_TargetTypeRon : Rounding  Operator=round
  ACC_TargetType_1sat : Saturate  UpperLimit=7  LowerLimit=0
  ACC_TargetType_Convert : DataTypeConversion  OutDataTypeStr=uint8
  ACC_TargetType_Convert1 : DataTypeConversion  OutDataTypeStr=uint32
  ACC_TargetType_D : Product  Inputs=*/
  ACC_TargetType_F : Constant  OutDataTypeStr=single
  ACC_TargetType_L : simulink/Logic and Bit Operations/Bitwise Operator  logicop=AND  UseBitMask=on  BitMask=7  BitMaskRealWorld=Stored Integer
  ACC_TargetType_O : Constant  Value=0  OutDataTypeStr=single
  ACC_TargetType_S : ArithShift
  ACC_TargetType_sat : Saturate  UpperLimit=0  LowerLimit=0
  ACC_TargetType_st : Sum  Inputs=+-
  Constant{1..3,5..8} (7 alike) : Constant  Value=0  OutDataTypeStr=uint8
  output1 : Outport
  output2 : Outport  Port=2
  output3 : Outport  Port=3
  output4 : Outport  Port=4
  output5 : Outport  Port=5
  output6 : Outport  Port=6
  output7 : Outport  Port=7
  output8 : Outport  Port=8
  wires:
  ACC_TargetType/1 -> ACC_TargetType_sat/1
  ACC_TargetType_sat/1 -> ACC_TargetType_st/1
  ACC_TargetType_O/1 -> ACC_TargetType_st/2
  ACC_TargetType_st/1 -> ACC_TargetType_D/1
  ACC_TargetType_F/1 -> ACC_TargetType_D/2
  ACC_TargetType_D/1 -> ACC_TargetTypeRon/1
  ACC_TargetTypeRon/1 -> ACC_TargetType_S/1
  ACC_TargetType_S/1 -> ACC_TargetType_1sat/1
  ACC_TargetType_1sat/1 -> ACC_TargetType_Convert1/1
  ACC_TargetType_Convert1/1 -> ACC_TargetType_L/1
  ACC_TargetType_L/1 -> ACC_TargetType_Convert/1
  ACC_TargetType_Convert/1 -> output4/1
  Constant1/1 -> output1/1
  Constant2/1 -> output2/1
  Constant3/1 -> output3/1
  Constant5/1 -> output5/1
  Constant6/1 -> output6/1
  Constant7/1 -> output7/1
  Constant8/1 -> output8/1

== system VCU_CS75_12_27_test_log/长安CS75底盘程序，20ms一次/Output/Subsystem/TransmitMessages2/ACC_3C5/CRC ==
  CRC : Inport
  CRCRon : Rounding  Operator=round
  CRC_1sat : Saturate  UpperLimit=255  LowerLimit=0
  CRC_Convert : DataTypeConversion  OutDataTypeStr=uint8
  CRC_Convert1 : DataTypeConversion  OutDataTypeStr=uint32
  CRC_D : Product  Inputs=*/
  CRC_F : Constant  OutDataTypeStr=single
  CRC_L : simulink/Logic and Bit Operations/Bitwise Operator  logicop=AND  UseBitMask=on  BitMask=255  BitMaskRealWorld=Stored Integer
  CRC_O : Constant  Value=0  OutDataTypeStr=single
  CRC_S : ArithShift
  CRC_sat : Saturate  UpperLimit=0  LowerLimit=0
  CRC_st : Sum  Inputs=+-
  Constant{1..7} (7 alike) : Constant  Value=0  OutDataTypeStr=uint8
  output1 : Outport
  output2 : Outport  Port=2
  output3 : Outport  Port=3
  output4 : Outport  Port=4
  output5 : Outport  Port=5
  output6 : Outport  Port=6
  output7 : Outport  Port=7
  output8 : Outport  Port=8
  wires:
  CRC/1 -> CRC_sat/1
  CRC_sat/1 -> CRC_st/1
  CRC_O/1 -> CRC_st/2
  CRC_st/1 -> CRC_D/1
  CRC_F/1 -> CRC_D/2
  CRC_D/1 -> CRCRon/1
  CRCRon/1 -> CRC_S/1
  CRC_S/1 -> CRC_1sat/1
  CRC_1sat/1 -> CRC_Convert1/1
  CRC_Convert1/1 -> CRC_L/1
  CRC_L/1 -> CRC_Convert/1
  CRC_Convert/1 -> output8/1
  Constant1/1 -> output1/1
  Constant2/1 -> output2/1
  Constant3/1 -> output3/1
  Constant4/1 -> output4/1
  Constant5/1 -> output5/1
  Constant6/1 -> output6/1
  Constant7/1 -> output7/1

== system VCU_CS75_12_27_test_log/长安CS75底盘程序，20ms一次/Output/Subsystem/TransmitMessages2/ACC_3C5/RollingConter ==
  RollingConter : Inport
  Constant{1..6,8} (7 alike) : Constant  Value=0  OutDataTypeStr=uint8
  RollingConterRon : Rounding  Operator=round
  RollingConter_1sat : Saturate  UpperLimit=15  LowerLimit=0
  RollingConter_Convert : DataTypeConversion  OutDataTypeStr=uint8
  RollingConter_Convert1 : DataTypeConversion  OutDataTypeStr=uint32
  RollingConter_D : Product  Inputs=*/
  RollingConter_F : Constant  OutDataTypeStr=single
  RollingConter_L : simulink/Logic and Bit Operations/Bitwise Operator  logicop=AND  UseBitMask=on  BitMask=15  BitMaskRealWorld=Stored Integer
  RollingConter_O : Constant  Value=0  OutDataTypeStr=single
  RollingConter_S : ArithShift
  RollingConter_sat : Saturate  UpperLimit=15  LowerLimit=0
  RollingConter_st : Sum  Inputs=+-
  output1 : Outport
  output2 : Outport  Port=2
  output3 : Outport  Port=3
  output4 : Outport  Port=4
  output5 : Outport  Port=5
  output6 : Outport  Port=6
  output7 : Outport  Port=7
  output8 : Outport  Port=8
  wires:
  RollingConter/1 -> RollingConter_sat/1
  RollingConter_sat/1 -> RollingConter_st/1
  RollingConter_O/1 -> RollingConter_st/2
  RollingConter_st/1 -> RollingConter_D/1
  RollingConter_F/1 -> RollingConter_D/2
  RollingConter_D/1 -> RollingConterRon/1
  RollingConterRon/1 -> RollingConter_S/1
  RollingConter_S/1 -> RollingConter_1sat/1
  RollingConter_1sat/1 -> RollingConter_Convert1/1
  RollingConter_Convert1/1 -> RollingConter_L/1
  RollingConter_L/1 -> RollingConter_Convert/1
  RollingConter_Convert/1 -> output7/1
  Constant1/1 -> output1/1
  Constant2/1 -> output2/1
  Constant3/1 -> output3/1
  Constant4/1 -> output4/1
  Constant5/1 -> output5/1
  Constant6/1 -> output6/1
  Constant8/1 -> output8/1

== system VCU_CS75_12_27_test_log/长安CS75底盘程序，20ms一次/Output/Subsystem/TransmitMessages3/ACC_3D5/ACC_LeftTargetDection ==
  ACC_LeftTargetDection : Inport
  ACC_LeftTargetDectionRon : Rounding  Operator=round
  ACC_LeftTargetDection_1sat : Saturate  UpperLimit=24  LowerLimit=0
  ACC_LeftTargetDection_Convert : DataTypeConversion  OutDataTypeStr=uint8
  ACC_LeftTargetDection_Convert1 : DataTypeConversion  OutDataTypeStr=uint32
  ACC_LeftTargetDection_D : Product  Inputs=*/
  ACC_LeftTargetDection_F : Constant  OutDataTypeStr=single
  ACC_LeftTargetDection_L : simulink/Logic and Bit Operations/Bitwise Operator  logicop=AND  UseBitMask=on  BitMask=24  BitMaskRealWorld=Stored Integer
  ACC_LeftTargetDection_O : Constant  Value=0  OutDataTypeStr=single
  ACC_LeftTargetDection_S : ArithShift  BitShiftNumber=-3
  ACC_LeftTargetDection_sat : Saturate  UpperLimit=0  LowerLimit=0
  ACC_LeftTargetDection_st : Sum  Inputs=+-
  Constant{2..8} (7 alike) : Constant  Value=0  OutDataTypeStr=uint8
  output1 : Outport
  output2 : Outport  Port=2
  output3 : Outport  Port=3
  output4 : Outport  Port=4
  output5 : Outport  Port=5
  output6 : Outport  Port=6
  output7 : Outport  Port=7
  output8 : Outport  Port=8
  wires:
  ACC_LeftTargetDection/1 -> ACC_LeftTargetDection_sat/1
  ACC_LeftTargetDection_sat/1 -> ACC_LeftTargetDection_st/1
  ACC_LeftTargetDection_O/1 -> ACC_LeftTargetDection_st/2
  ACC_LeftTargetDection_st/1 -> ACC_LeftTargetDection_D/1
  ACC_LeftTargetDection_F/1 -> ACC_LeftTargetDection_D/2
  ACC_LeftTargetDection_D/1 -> ACC_LeftTargetDectionRon/1
  ACC_LeftTargetDectionRon/1 -> ACC_LeftTargetDection_S/1
  ACC_LeftTargetDection_S/1 -> ACC_LeftTargetDection_1sat/1
  ACC_LeftTargetDection_1sat/1 -> ACC_LeftTargetDection_Convert1/1
  ACC_LeftTargetDection_Convert1/1 -> ACC_LeftTargetDection_L/1
  ACC_LeftTargetDection_L/1 -> ACC_LeftTargetDection_Convert/1
  ACC_LeftTargetDection_Convert/1 -> output1/1
  Constant2/1 -> output2/1
  Constant3/1 -> output3/1
  Constant4/1 -> output4/1
  Constant5/1 -> output5/1
  Constant6/1 -> output6/1
  Constant7/1 -> output7/1
  Constant8/1 -> output8/1

== system VCU_CS75_12_27_test_log/长安CS75底盘程序，20ms一次/Output/Subsystem/TransmitMessages3/ACC_3D5/ACC_LeftTargetLatRange ==
  ACC_LeftTargetLatRange : Inport
  ACC_LeftTargetLatRangeBitCov : DataTypeConversion  OutDataTypeStr=uint8
  ACC_LeftTargetLatRangeCOV : DataTypeConversion  OutDataTypeStr=uint8
  ACC_LeftTargetLatRangeRon : Rounding  Operator=round
  ACC_LeftTargetLatRange_1sat : Saturate  UpperLimit=8184  LowerLimit=0
  ACC_LeftTargetLatRange_And : simulink/Logic and Bit Operations/Bitwise Operator  logicop=AND  UseBitMask=off  NumInputPorts=2  BitMask=bin2dec('11011001')  BitMaskRealWorld=Stored Integer
  ACC_LeftTargetLatRange_And_C : Constant  Value=255  OutDataTypeStr=uint32
  ACC_LeftTargetLatRange_Convert : DataTypeConversion  OutDataTypeStr=uint32
  ACC_LeftTargetLatRange_D : Product  Inputs=*/
  ACC_LeftTargetLatRange_D1 : Product  Inputs=*/
  ACC_LeftTargetLatRange_F : Constant  Value=0.1  OutDataTypeStr=single
  ACC_LeftTargetLatRange_L : simulink/Logic and Bit Operations/Bitwise Operator  logicop=AND  UseBitMask=on  BitMask=8184  BitMaskRealWorld=Stored Integer
  ACC_LeftTargetLatRange_O : Constant  Value=-50  OutDataTypeStr=single
  ACC_LeftTargetLatRange_S : ArithShift  BitShiftNumber=-3
  ACC_LeftTargetLatRange_sat : Saturate  UpperLimit=0  LowerLimit=0
  ACC_LeftTargetLatRange_st : Sum  Inputs=+-
  ACC_LeftTargetLatRangeoutput3_C : Constant  Value=256
  Constant{1..2,5..8} (6 alike) : Constant  Value=0  OutDataTypeStr=uint8
  output1 : Outport
  output2 : Outport  Port=2
  output3 : Outport  Port=3
  output4 : Outport  Port=4
  output5 : Outport  Port=5
  output6 : Outport  Port=6
  output7 : Outport  Port=7
  output8 : Outport  Port=8
  wires:
  ACC_LeftTargetLatRange/1 -> ACC_LeftTargetLatRange_sat/1
  ACC_LeftTargetLatRange_sat/1 -> ACC_LeftTargetLatRange_st/1
  ACC_LeftTargetLatRange_O/1 -> ACC_LeftTargetLatRange_st/2
  ACC_LeftTargetLatRange_st/1 -> ACC_LeftTargetLatRange_D/1
  ACC_LeftTargetLatRange_F/1 -> ACC_LeftTargetLatRange_D/2
  ACC_LeftTargetLatRange_D/1 -> ACC_LeftTargetLatRangeRon/1
  ACC_LeftTargetLatRangeRon/1 -> ACC_LeftTargetLatRange_S/1
  ACC_LeftTargetLatRange_S/1 -> ACC_LeftTargetLatRange_1sat/1
  ACC_LeftTargetLatRange_1sat/1 -> ACC_LeftTargetLatRange_Convert/1
  ACC_LeftTargetLatRange_Convert/1 -> ACC_LeftTargetLatRange_L/1
  ACC_LeftTargetLatRange_L/1 -> ACC_LeftTargetLatRange_D1/1, ACC_LeftTargetLatRange_And/1
  ACC_LeftTargetLatRangeoutput3_C/1 -> ACC_LeftTargetLatRange_D1/2
  ACC_LeftTargetLatRange_D1/1 -> ACC_LeftTargetLatRangeCOV/1
  ACC_LeftTargetLatRangeCOV/1 -> output3/1
  ACC_LeftTargetLatRange_And_C/1 -> ACC_LeftTargetLatRange_And/2
  ACC_LeftTargetLatRange_And/1 -> ACC_LeftTargetLatRangeBitCov/1
  ACC_LeftTargetLatRangeBitCov/1 -> output4/1
  Constant1/1 -> output1/1
  Constant2/1 -> output2/1
  Constant5/1 -> output5/1
  Constant6/1 -> output6/1
  Constant7/1 -> output7/1
  Constant8/1 -> output8/1

== system VCU_CS75_12_27_test_log/长安CS75底盘程序，20ms一次/Output/Subsystem/TransmitMessages3/ACC_3D5/ACC_LeftTargetLngRange ==
  ACC_LeftTargetLngRange : Inport
  ACC_LeftTargetLngRangeBitCov : DataTypeConversion  OutDataTypeStr=uint8
  ACC_LeftTargetLngRangeCOV : DataTypeConversion  OutDataTypeStr=uint8
  ACC_LeftTargetLngRangeRon : Rounding  Operator=round
  ACC_LeftTargetLngRange_1sat : Saturate  UpperLimit=511  LowerLimit=0
  ACC_LeftTargetLngRange_And : simulink/Logic and Bit Operations/Bitwise Operator  logicop=AND  UseBitMask=off  NumInputPorts=2  BitMask=bin2dec('11011001')  BitMaskRealWorld=Stored Integer
  ACC_LeftTargetLngRange_And_C : Constant  Value=255  OutDataTypeStr=uint32
  ACC_LeftTargetLngRange_Convert : DataTypeConversion  OutDataTypeStr=uint32
  ACC_LeftTargetLngRange_D : Product  Inputs=*/
  ACC_LeftTargetLngRange_D1 : Product  Inputs=*/
  ACC_LeftTargetLngRange_F : Constant  Value=0.5  OutDataTypeStr=single
  ACC_LeftTargetLngRange_L : simulink/Logic and Bit Operations/Bitwise Operator  logicop=AND  UseBitMask=on  BitMask=511  BitMaskRealWorld=Stored Integer
  ACC_LeftTargetLngRange_O : Constant  Value=0  OutDataTypeStr=single
  ACC_LeftTargetLngRange_S : ArithShift
  ACC_LeftTargetLngRange_sat : Saturate  UpperLimit=0  LowerLimit=0
  ACC_LeftTargetLngRange_st : Sum  Inputs=+-
  ACC_LeftTargetLngRangeoutput1_C : Constant  Value=256
  Constant{3..8} (6 alike) : Constant  Value=0  OutDataTypeStr=uint8
  output1 : Outport
  output2 : Outport  Port=2
  output3 : Outport  Port=3
  output4 : Outport  Port=4
  output5 : Outport  Port=5
  output6 : Outport  Port=6
  output7 : Outport  Port=7
  output8 : Outport  Port=8
  wires:
  ACC_LeftTargetLngRange/1 -> ACC_LeftTargetLngRange_sat/1
  ACC_LeftTargetLngRange_sat/1 -> ACC_LeftTargetLngRange_st/1
  ACC_LeftTargetLngRange_O/1 -> ACC_LeftTargetLngRange_st/2
  ACC_LeftTargetLngRange_st/1 -> ACC_LeftTargetLngRange_D/1
  ACC_LeftTargetLngRange_F/1 -> ACC_LeftTargetLngRange_D/2
  ACC_LeftTargetLngRange_D/1 -> ACC_LeftTargetLngRangeRon/1
  ACC_LeftTargetLngRangeRon/1 -> ACC_LeftTargetLngRange_S/1
  ACC_LeftTargetLngRange_S/1 -> ACC_LeftTargetLngRange_1sat/1
  ACC_LeftTargetLngRange_1sat/1 -> ACC_LeftTargetLngRange_Convert/1
  ACC_LeftTargetLngRange_Convert/1 -> ACC_LeftTargetLngRange_L/1
  ACC_LeftTargetLngRange_L/1 -> ACC_LeftTargetLngRange_D1/1, ACC_LeftTargetLngRange_And/1
  ACC_LeftTargetLngRangeoutput1_C/1 -> ACC_LeftTargetLngRange_D1/2
  ACC_LeftTargetLngRange_D1/1 -> ACC_LeftTargetLngRangeCOV/1
  ACC_LeftTargetLngRangeCOV/1 -> output1/1
  ACC_LeftTargetLngRange_And_C/1 -> ACC_LeftTargetLngRange_And/2
  ACC_LeftTargetLngRange_And/1 -> ACC_LeftTargetLngRangeBitCov/1
  ACC_LeftTargetLngRangeBitCov/1 -> output2/1
  Constant3/1 -> output3/1
  Constant4/1 -> output4/1
  Constant5/1 -> output5/1
  Constant6/1 -> output6/1
  Constant7/1 -> output7/1
  Constant8/1 -> output8/1
